simulink model "Simulacao_Exemplo_2C"  (R2015a)
settings: Solver=ode45  StartTime=0.0  StopTime=240  FixedStep=0.1  MaxStep=5e-1  RelTol=1e-3
libraries: simulink x6
settings Model: CovSFcnEnable=off  Creator=MeneghettiAir  LastModifiedBy=QG
settings DebuggingCC: SolverPrmCheckMsg=warning

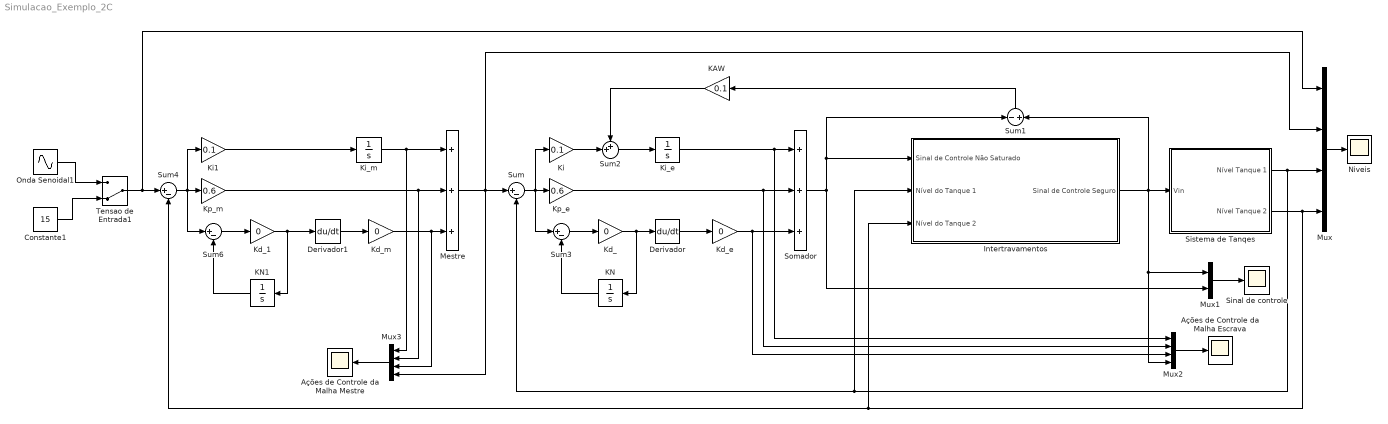
== system Simulacao_Exemplo_2C ==
  Ações de Controle da Malha Escrava : Scope
      settings: ShowLegends=on  TimeRange=240  YMax=35  SaveName=S_Controle1  MaxDataPoints=500000
  Ações de Controle da Malha Mestre : Scope
      settings: ShowLegends=on  TimeRange=240  YMax=35  SaveName=S_Controle2  MaxDataPoints=500000
  Constante1 : Constant  Value=15
  Derivador : Derivative
  Derivador1 : Derivative
  Intertravamentos : Subsystem
  KAW : Gain  Gain=0.1
  KN : Integrator
  KN1 : Integrator
  Kd_ : Gain  Gain=0
  Kd_1 : Gain  Gain=0
  Kd_e : Gain  Gain=0
  Kd_m : Gain  Gain=0
  Ki : Gain  Gain=0.1
  Ki1 : Gain  Gain=0.1
  Ki_e : Integrator
  Ki_m : Integrator
  Kp_e : Gain  Gain=0.6
  Kp_m : Gain  Gain=0.6
  Mestre : Sum  Inputs=+++
  Mux : Mux
  Mux1 : Mux  Inputs=2
  Mux2 : Mux
  Mux3 : Mux
  Niveis : Scope
      settings: ShowLegends=on  TimeRange=240  YMax=35  SaveName=Niveis  MaxDataPoints=500000
  Onda Senoidal1 : Sin  Amplitude=2  Bias=14  Frequency=0.2  SampleTime=0
  Sinal de controle : Scope
      settings: ShowLegends=on  TimeRange=240  YMax=35  SaveName=S_Controle  MaxDataPoints=500000
  "Sistema de Tanqes " : Subsystem
  Somador : Sum  Inputs=+++
  Sum{,3..4,6} (4 alike) : Sum  Inputs=|+-
  Sum1 : Sum  Inputs=-|+
  Sum2 : Sum  Inputs=++|
  Tensao de Entrada1 : ManualSwitch  CurrentSetting=0
  wires:
  "Sistema de Tanqes "/2(Nível Tanque 2) -> Mux/4, Intertravamentos/3(Nível do Tanque 2), Sum4/2
  Mux/1 -> Niveis/1
  Mestre/1 -> Mux3/4, Mux/2, Sum/1
  Mux1/1 -> Sinal de controle/1
  Sum/1 -> Sum3/1, Ki/1, Kp_e/1
  Somador/1 -> Sum1/1, Intertravamentos/1(Sinal de Controle Não Saturado), Mux1/2
  Ki_e/1 -> Mux2/1, Somador/1
  Kp_e/1 -> Mux2/2, Somador/2
  Mux2/1 -> Ações de Controle da Malha Escrava/1
  Sum1/1 -> KAW/1
  KAW/1 -> Sum2/1
  Sum2/1 -> Ki_e/1
  Ki/1 -> Sum2/2
  Sum3/1 -> Kd_/1
  KN/1 -> Sum3/2
  Intertravamentos/1(Sinal de Controle Seguro) -> "Sistema de Tanqes "/1(Vin), Mux1/1, Mux2/4, Sum1/2
  "Sistema de Tanqes "/1(Nível Tanque 1) -> Mux/3, Sum/2, Intertravamentos/2(Nível do Tanque 1)
  Tensao de Entrada1/1 -> Mux/1, Sum4/1
  Constante1/1 -> Tensao de Entrada1/2
  Onda Senoidal1/1 -> Tensao de Entrada1/1
  Sum4/1 -> Sum6/1, Ki1/1, Kp_m/1
  Ki_m/1 -> Mux3/1, Mestre/1
  Kp_m/1 -> Mux3/2, Mestre/2
  Ki1/1 -> Ki_m/1
  Sum6/1 -> Kd_1/1
  KN1/1 -> Sum6/2
  Mux3/1 -> Ações de Controle da Malha Mestre/1
  Kd_e/1 -> Mux2/3, Somador/3
  Derivador/1 -> Kd_e/1
  Kd_/1 -> KN/1, Derivador/1
  Kd_1/1 -> KN1/1, Derivador1/1
  Kd_m/1 -> Mux3/3, Mestre/3
  Derivador1/1 -> Kd_m/1

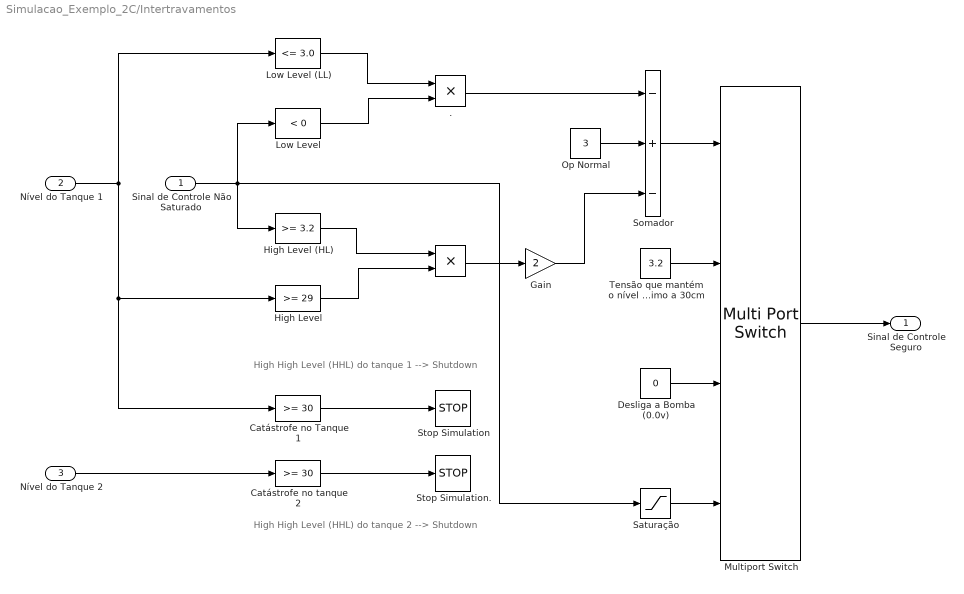
== system Simulacao_Exemplo_2C/Intertravamentos ==
  note: High High Level (HHL) do tanque 1 --> Shutdown
  note: High High Level (HHL) do tanque 2 --> Shutdown
  Sinal de Controle Não Saturado : Inport
  Nível do Tanque 1 : Inport  Port=2
  Nível do Tanque 2 : Inport  Port=3
  " " : Product
  . : Product
  Catástrofe no Tanque 1 : simulink/Logic and Bit Operations/Compare To Constant  relop=>=  const=30  OutDataTypeStr=boolean
  Catástrofe no tanque 2 : simulink/Logic and Bit Operations/Compare To Constant  relop=>=  const=30  OutDataTypeStr=boolean
  Desliga a Bomba (0.0v) : Constant  Value=0
  Gain : Gain  Gain=2
  High Level : simulink/Logic and Bit Operations/Compare To Constant  relop=>=  const=29  OutDataTypeStr=boolean
  High Level (HL) : simulink/Logic and Bit Operations/Compare To Constant  relop=>=  const=3.2  OutDataTypeStr=boolean
  Low Level : simulink/Logic and Bit Operations/Compare To Constant  relop=<  const=0  OutDataTypeStr=boolean
  Low Level (LL) : simulink/Logic and Bit Operations/Compare To Constant  relop=<=  const=3.0  OutDataTypeStr=boolean
  Multiport Switch : MultiPortSwitch
  Op Normal : Constant  Value=3
  Saturação : Saturate  UpperLimit=4  LowerLimit=-4
  Somador : Sum  Inputs=-+-
  Stop Simulation : Stop
  Stop Simulation. : Stop
  Tensão que mantém o nível próximo a 30cm : Constant  Value=3.2
  Sinal de Controle Seguro : Outport
  wires:
  Multiport Switch/1 -> Sinal de Controle Seguro/1
  Saturação/1 -> Multiport Switch/4
  Nível do Tanque 1/1 -> Catástrofe no Tanque 1/1, High Level/1, Low Level (LL)/1
  Sinal de Controle Não Saturado/1 -> High Level (HL)/1, Saturação/1, Low Level/1
  Desliga a Bomba (0.0v)/1 -> Multiport Switch/3
  Tensão que mantém o nível próximo a 30cm/1 -> Multiport Switch/2
  Somador/1 -> Multiport Switch/1
  Op Normal/1 -> Somador/2
  ./1 -> Somador/1
  Low Level (LL)/1 -> ./1
  Low Level/1 -> ./2
  Gain/1 -> Somador/3
  " "/1 -> Gain/1
  High Level (HL)/1 -> " "/1
  High Level/1 -> " "/2
  Catástrofe no Tanque 1/1 -> Stop Simulation/1
  Catástrofe no tanque 2/1 -> Stop Simulation./1
  Nível do Tanque 2/1 -> Catástrofe no tanque 2/1

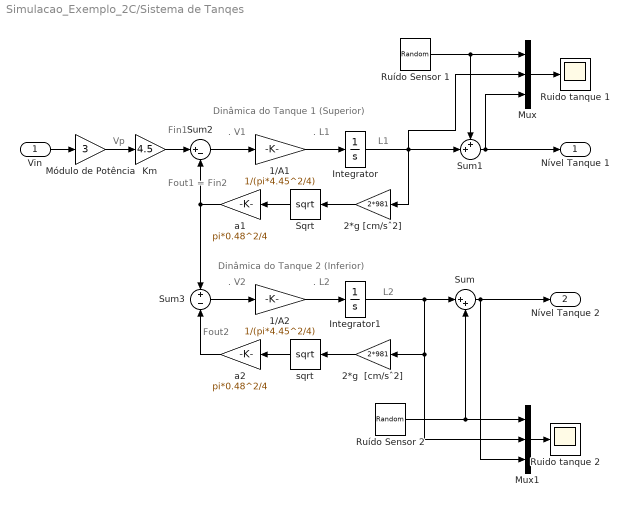
== system Simulacao_Exemplo_2C/Sistema de Tanqes  ==
  note: Dinâmica do Tanque 1 (Superior)
  note: L1
  note: Fin1
  note: Fout1
      | =
      | Fin2
  note: .
      | L1
  note: .
      | V1
  note: L2
  note: Fout2
  note: .
      | L2
  note: .
      | V2
  note: Dinâmica do Tanque 2 (Inferior)
  note: Vp
  Vin : Inport
  1/A1 : Gain  Gain=1/(pi*4.45^2/4)
  1/A2 : Gain  Gain=1/(pi*4.45^2/4)
  2*g  [cm/sˆ2] : Gain  Gain=2*981
  2*g [cm/sˆ2] : Gain  Gain=2*981
  Integrator : Integrator  UpperSaturationLimit=35  LowerSaturationLimit=-2
  Integrator1 : Integrator  UpperSaturationLimit=35  LowerSaturationLimit=-2
  Km : Gain  Gain=4.5
  Mux : Mux  Inputs=3
  Mux1 : Mux  Inputs=3
  Módulo de Potência : Gain  Gain=3
  Ruido tanque 1 : Scope
      settings: TimeRange=50  YMin=0  YMax=20  SaveName=ScopeData3
  Ruido tanque 2 : Scope
      settings: TimeRange=50  YMin=0  YMax=20  SaveName=ScopeData4
  Ruído Sensor 1 : UniformRandomNumber  Minimum=-0.0001  Maximum=0.0001  Seed=round(rand(1)*100)  SampleTime=0.5
  Ruído Sensor 2 : UniformRandomNumber  Minimum=-0.0001  Maximum=0.0001  Seed=round(rand(1)*100)  SampleTime=0.7
  Sqrt : Sqrt  SaturateOnIntegerOverflow=on
  Sum : Sum  Inputs=|++
  Sum1 : Sum  Inputs=++|
  Sum2 : Sum  Inputs=|+-
  Sum3 : Sum  Inputs=+-
  a1 : Gain  Gain=pi*0.48^2/4
  a2 : Gain  Gain=pi*0.48^2/4
  sqrt : Sqrt  SaturateOnIntegerOverflow=on
  Nível Tanque 1 : Outport
  Nível Tanque 2 : Outport  Port=2
  wires:
  Vin/1 -> Módulo de Potência/1
  Sum/1 -> Nível Tanque 2/1, Mux1/3
  Mux/1 -> Ruido tanque 1/1
  Mux1/1 -> Ruido tanque 2/1
  Sum1/1 -> Nível Tanque 1/1, Mux/3
  Ruído Sensor 1/1 -> Mux/1, Sum1/1
  Ruído Sensor 2/1 -> Sum/2, Mux1/1
  2*g [cm/sˆ2]/1 -> Sqrt/1
  Sqrt/1 -> a1/1
  Km/1 -> Sum2/1
  a1/1 -> Sum2/2, Sum3/1
  Sum2/1 -> 1/A1/1
  1/A1/1 -> Integrator/1
  2*g  [cm/sˆ2]/1 -> sqrt/1
  sqrt/1 -> a2/1
  Sum3/1 -> 1/A2/1
  1/A2/1 -> Integrator1/1
  a2/1 -> Sum3/2
  Módulo de Potência/1 -> Km/1
  Integrator/1 -> Sum1/2, Mux/2, 2*g [cm/sˆ2]/1
  Integrator1/1 -> Mux1/2, 2*g  [cm/sˆ2]/1, Sum/1
